simulink model "FLCSim3"  (R2019a)
settings: Solver=VariableStepAuto  StartTime=0.0  StopTime=18  MaxStep=0.01  RelTol=1e-4  EnableMultiTasking=on
undefined symbols (not defined in the file): sigbuilder_block
libraries: fuzblock x1
settings Model: SimulationMode=accelerator  Creator=Nikos  LastModifiedBy=gitop
settings DataIOCC: LimitDataPoints=on  SaveOutput=off  SaveTime=off  ReturnWorkspaceOutputs=off
settings OptimizationCC: ExpressionDepthLimit=2147483647  LifeSpan=1
settings DebuggingCC: UnderspecifiedInitializationDetection=Classic  MergeDetectMultiDrivingBlocksExec=none  FcnCallInpInsideContextMsg=warning  AllowSymbolicDim=off  StateNameClashWarn=warning  PregeneratedLibrarySubsystemCodeDiagnostic=none  SFUnexpectedBacktrackingDiag=warning  SFNoUnconditionalDefaultTransitionDiag=warning  SFExecutionAtInitializationDiag=none  ArithmeticOperatorsInVariantConditions=warning
settings SFSimCC: SimUseLocalCustomCode=off
settings RTWCC: RTWUseLocalCustomCode=off
settings CodeAppCC: StateflowObjectComments=on
settings GRTTargetCC: TargetLangStandard=C89/C90 (ANSI)  GeneratePreprocessorConditionals=Disable all  CombineOutputUpdateFcns=off  GRTInterface=on

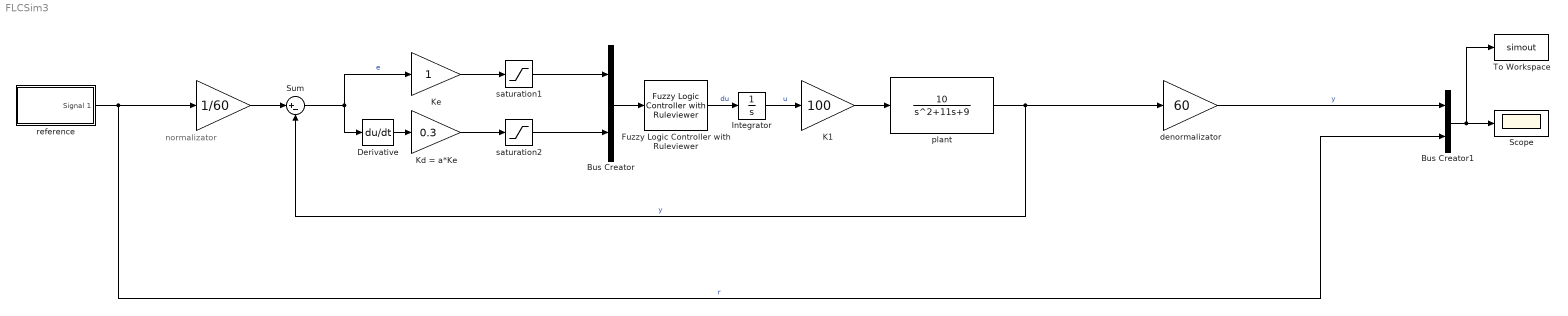
== system FLCSim3 ==
  note: normalizator
  " " : Gain  Gain=1/60
  " denormalizator" : Gain  Gain=60
  " Κ1" : Gain  Gain=100
  Bus Creator : BusCreator  Inputs=2
  Bus Creator1 : BusCreator  Inputs=2
  Derivative : Derivative
  Fuzzy Logic Controller with Ruleviewer : fuzblock/Fuzzy Logic  Controller  with Ruleviewer  fismatrix=FLC  Ts=.1
  Integrator : Integrator
  Kd = a*Ke : Gain  Gain=0.3
  Ke : Gain
  Scope : Scope
  Sum : Sum  Inputs=|+-
  To Workspace : ToWorkspace  VariableName=simout  SaveFormat=Structure With Time  SampleTime=-1
  plant : TransferFcn  Numerator=[10]  Denominator=[1 11 9]
  reference : Subsystem  Tag=STV Subsys  LoadFcn=sigbuilder_block('load');  StartFcn=sigbuilder_block('start');  StopFcn=sigbuilder_block('stop');  ClipboardFcn=sigbuilder_block('clipboard');  mask(Sigbuilder block){tuvar=[0:10]}
      mask help: Simulink:masks:SigbuilderBlock_MD
      mask init:
      | if ~strcmp(get_param(bdroot(gcbh),'SimulationStatus'),'stopped') tuvar = sigbuilder_block('maskInit'); end
      settings: CopyFcn=sigbuilder_block('copy');  DeleteFcn=sigbuilder_block('delete');  ModelCloseFcn=sigbuilder_block('modelClose');  PreSaveFcn=sigbuilder_block('preSave');  PauseFcn=sigbuilder_block('pause');  ContinueFcn=sigbuilder_block('continue');  NameChangeFcn=sigbuilder_block('namechange');  OpenFcn=sigbuilder_block('open',[448 38 478 405.5 ]);  CloseFcn=sigbuilder_block('close');
      mask Display: plot(0, 0, 100, 100,[2, 2, 32, 32, 2], [68, 8, 8, 68, 68],[32, 2], [38, 38], [32, 19, 2],[53, 60, 44], [32, 17, 17, 2],[16, 16, 31, 31]);txt = getActiveGroup(gcbh);text(2, 100, txt,'verticalAlignment', 'top');
  saturation1 : Saturate  UpperLimit=0.99  LowerLimit=-0.99
  saturation2 : Saturate  UpperLimit=0.99  LowerLimit=-0.99
  wires:
  plant/1 -> " denormalizator"/1, Sum/2  "y"
  reference/1(Signal 1) -> Bus Creator1/2, " "/1  "r"
  Fuzzy Logic Controller with Ruleviewer/1 -> Integrator/1  "du"
  Bus Creator/1 -> Fuzzy Logic Controller with Ruleviewer/1
  Ke/1 -> saturation1/1
  Sum/1 -> Derivative/1, Ke/1  "e"
  Derivative/1 -> Kd = a*Ke/1
  saturation2/1 -> Bus Creator/2
  " "/1 -> Sum/1
  Integrator/1 -> " Κ1"/1  "u"
  saturation1/1 -> Bus Creator/1
  Kd = a*Ke/1 -> saturation2/1
  " denormalizator"/1 -> Bus Creator1/1  "y"
  " Κ1"/1 -> plant/1
  Bus Creator1/1 -> To Workspace/1, Scope/1

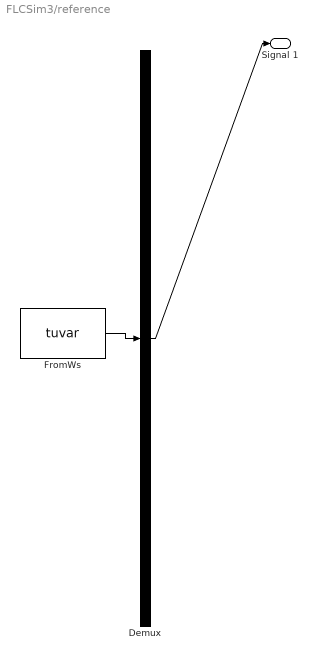
== system FLCSim3/reference ==
  Demux : Demux  Tag=STV Demux  Outputs=1
  FromWs : FromWorkspace  Tag=STV FromWs  VariableName=tuvar  SampleTime=0
      SigBuilderData=|
      | common.afterFinalStr = 'Extrapolate'
      | common.sampleTime = 0
      | dataSet.timeRange = [0 18]
      | dataSet.name = 'Group 1'
      | sbobj.Groups.Name = 'Group 1'
      | sbobj.Groups.Signals.Name = 'Signal 1'
      | sbobj.Groups.Signals.XData = [0 5 8 16 18]
      | sbobj.Groups.Signals.YData = [0 60 60 0 0]
      | sbobj.Groups.TimeRange = [0 18]
  Signal 1 : Outport  Tag=STV Outport
  wires:
  FromWs/1 -> Demux/1
  Demux/1 -> Signal 1/1
